simulink model "DBX_eARC_20220411_1632"  (R2021a)
settings: Solver=FixedStepAuto  StartTime=0.0  StopTime=inf  FixedStep=Ts  RelTol=1e-3  EnableMultiTasking=on
undefined symbols (not defined in the file): a, b, Cq, DiscIntNeverNeededParam, F_damper, Ff_spring, Fr_spring, FzF_0_w, FzR_0_w, h_CoG, h_RC, hs, hu, Ix, Iz, Kq, Kt, M, M_damp_f, M_damp_r, Mf_stiff, Mr_stiff, ms, mu, mui, params, theta_dot_f_damp, theta_dot_r_damp, theta_f_stiff, theta_r_stiff, tw, v_damper, Z_spring
libraries: CarMaker4SL x37, simulink_extras x1, simulink x1
(part 2 of 3)

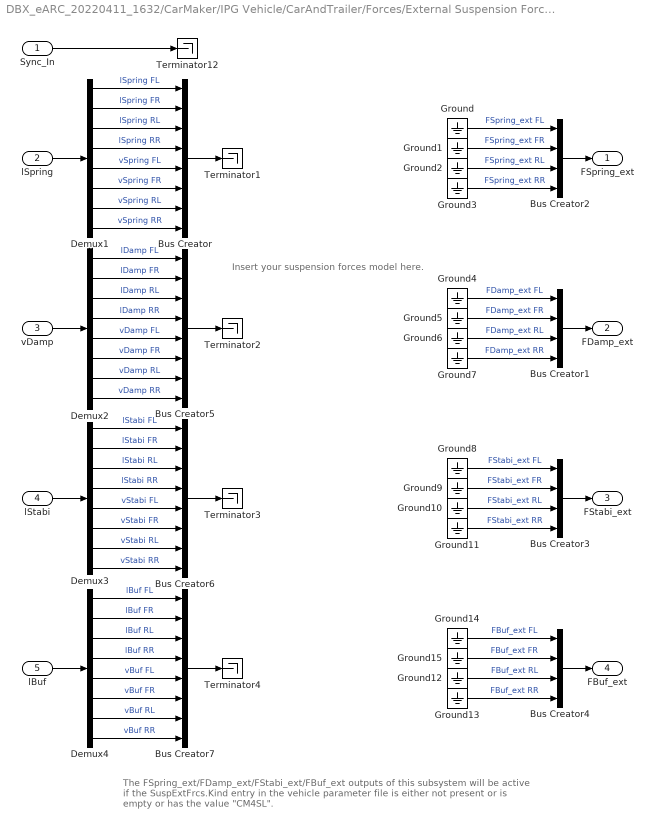
== system DBX_eARC_20220411_1632/CarMaker/IPG Vehicle/CarAndTrailer/Forces/External Suspension Forces ==
  note: The FSpring_ext/FDamp_ext/FStabi_ext/FBuf_ext outputs of this subsystem will be
      | active if the SuspExtFrcs.Kind entry in the vehicle parameter file
      | is either not present or is empty or has the value "CM4SL".
  note: Insert your suspension forces model here.
  Sync_In : Inport
  lSpring : Inport  Port=2
  vDamp : Inport  Port=3
  lStabi : Inport  Port=4
  lBuf : Inport  Port=5
  Bus Creator{,5..7} (4 alike) : BusCreator  Inputs=8
  Bus Creator{1..4} (4 alike) : BusCreator  Inputs=4
  Demux{1..4} (4 alike) : Demux  Outputs=8
      settings: DisplayOption=none
  Ground{,1..15} (16 alike) : Ground
  Terminator{1..4,12} (5 alike) : Terminator
  FSpring_ext : Outport
  FDamp_ext : Outport  Port=2
  FStabi_ext : Outport  Port=3
  FBuf_ext : Outport  Port=4
  wires:
  Bus Creator7/1 -> Terminator4/1
  Bus Creator6/1 -> Terminator3/1
  Bus Creator5/1 -> Terminator2/1
  Bus Creator/1 -> Terminator1/1
  Demux4/8 -> Bus Creator7/8  "vBuf RR"
  Demux4/7 -> Bus Creator7/7  "vBuf RL"
  Demux4/6 -> Bus Creator7/6  "vBuf FR"
  Demux4/5 -> Bus Creator7/5  "vBuf FL"
  Demux3/8 -> Bus Creator6/8  "vStabi RR"
  Demux3/7 -> Bus Creator6/7  "vStabi RL"
  Demux3/6 -> Bus Creator6/6  "vStabi FR"
  Demux3/5 -> Bus Creator6/5  "vStabi FL"
  Demux2/8 -> Bus Creator5/8  "vDamp RR"
  Demux2/7 -> Bus Creator5/7  "vDamp RL"
  Demux2/6 -> Bus Creator5/6  "vDamp FR"
  Demux2/5 -> Bus Creator5/5  "vDamp FL"
  Demux1/8 -> Bus Creator/8  "vSpring RR"
  Demux1/7 -> Bus Creator/7  "vSpring RL"
  Demux1/6 -> Bus Creator/6  "vSpring FR"
  Demux1/5 -> Bus Creator/5  "vSpring FL"
  Demux2/4 -> Bus Creator5/4  "lDamp RR"
  Demux2/3 -> Bus Creator5/3  "lDamp RL"
  Demux2/2 -> Bus Creator5/2  "lDamp FR"
  Demux2/1 -> Bus Creator5/1  "lDamp FL"
  Demux1/4 -> Bus Creator/4  "lSpring RR"
  Demux1/3 -> Bus Creator/3  "lSpring RL"
  Demux1/2 -> Bus Creator/2  "lSpring FR"
  Demux1/1 -> Bus Creator/1  "lSpring FL"
  Demux3/4 -> Bus Creator6/4  "lStabi RR"
  Demux3/3 -> Bus Creator6/3  "lStabi RL"
  Demux3/2 -> Bus Creator6/2  "lStabi FR"
  Demux3/1 -> Bus Creator6/1  "lStabi FL"
  lStabi/1 -> Demux3/1
  vDamp/1 -> Demux2/1
  lSpring/1 -> Demux1/1
  Demux4/4 -> Bus Creator7/4  "lBuf RR"
  Demux4/3 -> Bus Creator7/3  "lBuf RL"
  Demux4/2 -> Bus Creator7/2  "lBuf FR"
  Demux4/1 -> Bus Creator7/1  "lBuf FL"
  lBuf/1 -> Demux4/1
  Ground14/1 -> Bus Creator4/1  "FBuf_ext FL"
  Ground15/1 -> Bus Creator4/2  "FBuf_ext FR"
  Ground12/1 -> Bus Creator4/3  "FBuf_ext RL"
  Ground13/1 -> Bus Creator4/4  "FBuf_ext RR"
  Bus Creator4/1 -> FBuf_ext/1
  Sync_In/1 -> Terminator12/1
  Bus Creator2/1 -> FSpring_ext/1
  Ground/1 -> Bus Creator2/1  "FSpring_ext FL"
  Ground1/1 -> Bus Creator2/2  "FSpring_ext FR"
  Ground2/1 -> Bus Creator2/3  "FSpring_ext RL"
  Ground3/1 -> Bus Creator2/4  "FSpring_ext RR"
  Ground4/1 -> Bus Creator1/1  "FDamp_ext FL"
  Ground5/1 -> Bus Creator1/2  "FDamp_ext FR"
  Ground6/1 -> Bus Creator1/3  "FDamp_ext RL"
  Ground7/1 -> Bus Creator1/4  "FDamp_ext RR"
  Bus Creator1/1 -> FDamp_ext/1
  Ground8/1 -> Bus Creator3/1  "FStabi_ext FL"
  Ground9/1 -> Bus Creator3/2  "FStabi_ext FR"
  Ground10/1 -> Bus Creator3/3  "FStabi_ext RL"
  Ground11/1 -> Bus Creator3/4  "FStabi_ext RR"
  Bus Creator3/1 -> FStabi_ext/1

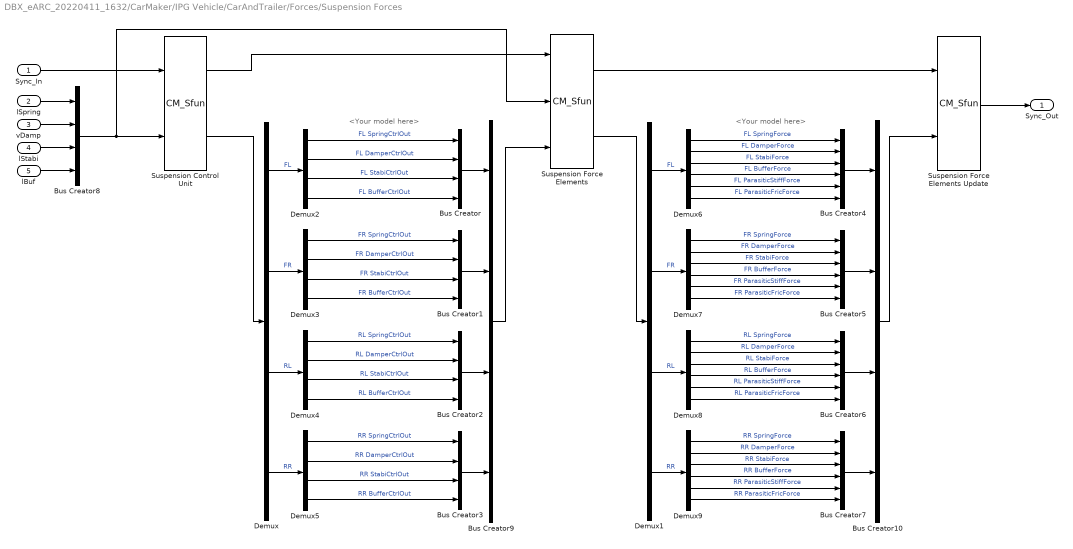
== system DBX_eARC_20220411_1632/CarMaker/IPG Vehicle/CarAndTrailer/Forces/Suspension Forces ==
  note: <Your model here>
  note: <Your model here>
  Sync_In : Inport
  lSpring : Inport  Port=2
  vDamp : Inport  Port=3
  lStabi : Inport  Port=4
  lBuf : Inport  Port=5
  Bus Creator{,1..3,8..10} (7 alike) : BusCreator  Inputs=4
  Bus Creator{4..7} (4 alike) : BusCreator  Inputs=6
  Demux{,1..5} (6 alike) : Demux
  Demux{6..9} (4 alike) : Demux  Outputs=6
  Suspension Control Unit : S-Function  FunctionName=CM_Sfun  Parameters='ForcesSuspControl'  SFunctionDeploymentMode=off  EnableBusSupport=off
  Suspension Force Elements : S-Function  FunctionName=CM_Sfun  Parameters='ForcesSusp'  SFunctionDeploymentMode=off  EnableBusSupport=off
  Suspension Force Elements Update : S-Function  FunctionName=CM_Sfun  Parameters='ForcesSuspUpd'  SFunctionDeploymentMode=off  EnableBusSupport=off
  Sync_Out : Outport
  wires:
  vDamp/1 -> Bus Creator8/2
  lStabi/1 -> Bus Creator8/3
  lBuf/1 -> Bus Creator8/4
  lSpring/1 -> Bus Creator8/1
  Bus Creator8/1 -> Suspension Control Unit/2, Suspension Force Elements/2
  Sync_In/1 -> Suspension Control Unit/1
  Suspension Control Unit/1 -> Suspension Force Elements/1
  Suspension Force Elements/1 -> Suspension Force Elements Update/1
  Suspension Force Elements Update/1 -> Sync_Out/1
  Bus Creator4/1 -> Bus Creator10/1
  Bus Creator5/1 -> Bus Creator10/2
  Bus Creator6/1 -> Bus Creator10/3
  Bus Creator7/1 -> Bus Creator10/4
  Demux6/1 -> Bus Creator4/1  "FL SpringForce"
  Demux9/1 -> Bus Creator7/1  "RR SpringForce"
  Demux9/2 -> Bus Creator7/2  "RR DamperForce"
  Demux9/3 -> Bus Creator7/3  "RR StabiForce"
  Demux9/4 -> Bus Creator7/4  "RR BufferForce"
  Demux9/5 -> Bus Creator7/5  "RR ParasiticStiffForce"
  Demux9/6 -> Bus Creator7/6  "RR ParasiticFricForce"
  Demux8/1 -> Bus Creator6/1  "RL SpringForce"
  Demux8/2 -> Bus Creator6/2  "RL DamperForce"
  Demux8/4 -> Bus Creator6/4  "RL BufferForce"
  Demux8/5 -> Bus Creator6/5  "RL ParasiticStiffForce"
  Demux8/6 -> Bus Creator6/6  "RL ParasiticFricForce"
  Demux8/3 -> Bus Creator6/3  "RL StabiForce"
  Demux7/1 -> Bus Creator5/1  "FR SpringForce"
  Demux7/2 -> Bus Creator5/2  "FR DamperForce"
  Demux7/3 -> Bus Creator5/3  "FR StabiForce"
  Demux7/4 -> Bus Creator5/4  "FR BufferForce"
  Demux7/5 -> Bus Creator5/5  "FR ParasiticStiffForce"
  Demux7/6 -> Bus Creator5/6  "FR ParasiticFricForce"
  Demux6/2 -> Bus Creator4/2  "FL DamperForce"
  Demux6/3 -> Bus Creator4/3  "FL StabiForce"
  Demux6/4 -> Bus Creator4/4  "FL BufferForce"
  Demux6/5 -> Bus Creator4/5  "FL ParasiticStiffForce"
  Demux6/6 -> Bus Creator4/6  "FL ParasiticFricForce"
  Bus Creator10/1 -> Suspension Force Elements Update/2
  Demux/1 -> Demux2/1  "FL"
  Bus Creator1/1 -> Bus Creator9/2
  Demux/2 -> Demux3/1  "FR"
  Bus Creator2/1 -> Bus Creator9/3
  Demux/3 -> Demux4/1  "RL"
  Bus Creator3/1 -> Bus Creator9/4
  Demux2/1 -> Bus Creator/1  "FL SpringCtrlOut"
  Demux/4 -> Demux5/1  "RR"
  Demux5/1 -> Bus Creator3/1  "RR SpringCtrlOut"
  Demux5/2 -> Bus Creator3/2  "RR DamperCtrlOut"
  Demux5/3 -> Bus Creator3/3  "RR StabiCtrlOut"
  Demux5/4 -> Bus Creator3/4  "RR BufferCtrlOut"
  Demux4/1 -> Bus Creator2/1  "RL SpringCtrlOut"
  Demux4/2 -> Bus Creator2/2  "RL DamperCtrlOut"
  Demux4/4 -> Bus Creator2/4  "RL BufferCtrlOut"
  Demux4/3 -> Bus Creator2/3  "RL StabiCtrlOut"
  Demux3/1 -> Bus Creator1/1  "FR SpringCtrlOut"
  Demux3/2 -> Bus Creator1/2  "FR DamperCtrlOut"
  Demux3/3 -> Bus Creator1/3  "FR StabiCtrlOut"
  Demux3/4 -> Bus Creator1/4  "FR BufferCtrlOut"
  Demux2/2 -> Bus Creator/2  "FL DamperCtrlOut"
  Demux2/3 -> Bus Creator/3  "FL StabiCtrlOut"
  Demux2/4 -> Bus Creator/4  "FL BufferCtrlOut"
  Suspension Control Unit/2 -> Demux/1
  Bus Creator9/1 -> Suspension Force Elements/3
  Bus Creator/1 -> Bus Creator9/1
  Suspension Force Elements/2 -> Demux1/1
  Demux1/1 -> Demux6/1  "FL"
  Demux1/2 -> Demux7/1  "FR"
  Demux1/3 -> Demux8/1  "RL"
  Demux1/4 -> Demux9/1  "RR"

== system DBX_eARC_20220411_1632/CarMaker/IPG Vehicle/CarAndTrailer/Forces/Tires ==
  note: The TireXX_Out signals will only be used if FileIdent is "CarMaker-Tire-CM4SL" in the tire parameter file!
      | An example parameter file can be found in Data/Tire/DT_CM4SL_UserTire.
  Sync_In : Inport
  TireFL_In : Inport  Port=2
  TireFR_In : Inport  Port=3
  TireRL_In : Inport  Port=4
  TireRR_In : Inport  Port=5
  Bus Creator{1..4} (4 alike) : BusCreator  Inputs=11
  Demux{1..3,8} (4 alike) : Demux  Outputs=7
      settings: DisplayOption=none
  TireFL : Subsystem
  TireFR : Subsystem
  TireRL : Subsystem
  TireRR : Subsystem
  TireFL_Out : Outport
  TireFR_Out : Outport  Port=2
  TireRL_Out : Outport  Port=3
  TireRR_Out : Outport  Port=4
  wires:
  Sync_In/1 -> TireRR/1(Sync_In), TireRL/1(Sync_In), TireFR/1(Sync_In), TireFL/1(Sync_In)
  Bus Creator4/1 -> TireRR_Out/1
  Bus Creator2/1 -> TireRL_Out/1
  Bus Creator1/1 -> TireFR_Out/1
  Demux3/5 -> TireRR/6(Rim_turnv)  "Tire_In Rim_turnv"
  Demux3/4 -> TireRR/5(Rim_rotv)  "Tire_In Rim_rotv"
  Demux3/1 -> TireRR/2(Load)  "Tire_In Load"
  Demux3/7 -> TireRR/8(muRoad)  "Tire_In mu"
  Demux3/6 -> TireRR/7(InclinAngle)  "Tire_In Camber"
  Demux3/2 -> TireRR/3(vxtrans)  "Tire_In vxtrans"
  Demux3/3 -> TireRR/4(vytrans)  "Tire_In vytrans"
  TireRR/11(AlignTrq) -> Bus Creator4/11  "Tire_Out AlignTrq"
  TireRR/10(RollResist) -> Bus Creator4/10  "Tire_Out RollResist"
  TireRR/9(OverturnTrq) -> Bus Creator4/9  "Tire_Out OverturnTrq"
  TireRR/8(LoadFrc) -> Bus Creator4/8  "Tire_Out LoadFrc"
  TireRR/7(SideFrc) -> Bus Creator4/7  "Tire_Out SideFrc"
  TireRR/6(LongFrc) -> Bus Creator4/6  "Tire_Out LongFrc"
  TireRR/5(vBelt) -> Bus Creator4/5  "Tire_Out vBelt"
  TireRR/4(rBelt_eff) -> Bus Creator4/4  "Tire_Out rBelt_eff"
  TireRR/3(TurnSlp) -> Bus Creator4/3  "Tire_Out TurnSlp"
  TireRR/1(Slp) -> Bus Creator4/1  "Tire_Out Slp"
  TireRR/2(Alpha) -> Bus Creator4/2  "Tire_Out Alpha"
  Demux2/5 -> TireRL/6(Rim_turnv)  "Tire_In Rim_turnv"
  Demux2/4 -> TireRL/5(Rim_rotv)  "Tire_In Rim_rotv"
  Demux2/1 -> TireRL/2(Load)  "Tire_In Load"
  Demux2/7 -> TireRL/8(muRoad)  "Tire_In mu"
  Demux2/6 -> TireRL/7(InclinAngle)  "Tire_In Camber"
  Demux2/2 -> TireRL/3(vxtrans)  "Tire_In vxtrans"
  Demux2/3 -> TireRL/4(vytrans)  "Tire_In vytrans"
  TireRL/11(AlignTrq) -> Bus Creator2/11  "Tire_Out AlignTrq"
  TireRL/10(RollResist) -> Bus Creator2/10  "Tire_Out RollResist"
  TireRL/9(OverturnTrq) -> Bus Creator2/9  "Tire_Out OverturnTrq"
  TireRL/8(LoadFrc) -> Bus Creator2/8  "Tire_Out LoadFrc"
  TireRL/7(SideFrc) -> Bus Creator2/7  "Tire_Out SideFrc"
  TireRL/6(LongFrc) -> Bus Creator2/6  "Tire_Out LongFrc"
  TireRL/5(vBelt) -> Bus Creator2/5  "Tire_Out vBelt"
  TireRL/4(rBelt_eff) -> Bus Creator2/4  "Tire_Out rBelt_eff"
  TireRL/3(TurnSlp) -> Bus Creator2/3  "Tire_Out TurnSlp"
  TireRL/1(Slp) -> Bus Creator2/1  "Tire_Out Slp"
  TireRL/2(Alpha) -> Bus Creator2/2  "Tire_Out Alpha"
  Demux1/5 -> TireFR/6(Rim_turnv)  "Tire_In Rim_turnv"
  Demux1/4 -> TireFR/5(Rim_rotv)  "Tire_In Rim_rotv"
  Demux1/1 -> TireFR/2(Load)  "Tire_In Load"
  Demux1/7 -> TireFR/8(muRoad)  "Tire_In mu"
  Demux1/6 -> TireFR/7(InclinAngle)  "Tire_In Camber"
  Demux1/2 -> TireFR/3(vxtrans)  "Tire_In vxtrans"
  Demux1/3 -> TireFR/4(vytrans)  "Tire_In vytrans"
  TireFR/11(AlignTrq) -> Bus Creator1/11  "Tire_Out AlignTrq"
  TireFR/10(RollResist) -> Bus Creator1/10  "Tire_Out RollResist"
  TireFR/9(OverturnTrq) -> Bus Creator1/9  "Tire_Out OverturnTrq"
  TireFR/8(LoadFrc) -> Bus Creator1/8  "Tire_Out LoadFrc"
  TireFR/7(SideFrc) -> Bus Creator1/7  "Tire_Out SideFrc"
  TireFR/6(LongFrc) -> Bus Creator1/6  "Tire_Out LongFrc"
  TireFR/5(vBelt) -> Bus Creator1/5  "Tire_Out vBelt"
  TireFR/4(rBelt_eff) -> Bus Creator1/4  "Tire_Out rBelt_eff"
  TireFR/3(TurnSlp) -> Bus Creator1/3  "Tire_Out TurnSlp"
  TireFR/1(Slp) -> Bus Creator1/1  "Tire_Out Slp"
  TireFR/2(Alpha) -> Bus Creator1/2  "Tire_Out Alpha"
  Demux8/5 -> TireFL/6(Rim_turnv)  "Tire_In Rim_turnv"
  Demux8/4 -> TireFL/5(Rim_rotv)  "Tire_In Rim_rotv"
  TireFL_In/1 -> Demux8/1
  Demux8/1 -> TireFL/2(Load)  "Tire_In Load"
  Demux8/7 -> TireFL/8(muRoad)  "Tire_In mu"
  Demux8/6 -> TireFL/7(InclinAngle)  "Tire_In Camber"
  Demux8/2 -> TireFL/3(vxtrans)  "Tire_In vxtrans"
  Demux8/3 -> TireFL/4(vytrans)  "Tire_In vytrans"
  TireFL/11(AlignTrq) -> Bus Creator3/11  "Tire_Out AlignTrq"
  TireFL/10(RollResist) -> Bus Creator3/10  "Tire_Out RollResist"
  TireFL/9(OverturnTrq) -> Bus Creator3/9  "Tire_Out OverturnTrq"
  TireFL/8(LoadFrc) -> Bus Creator3/8  "Tire_Out LoadFrc"
  TireFL/7(SideFrc) -> Bus Creator3/7  "Tire_Out SideFrc"
  TireFL/6(LongFrc) -> Bus Creator3/6  "Tire_Out LongFrc"
  TireFL/5(vBelt) -> Bus Creator3/5  "Tire_Out vBelt"
  TireFL/4(rBelt_eff) -> Bus Creator3/4  "Tire_Out rBelt_eff"
  TireFL/3(TurnSlp) -> Bus Creator3/3  "Tire_Out TurnSlp"
  TireFL/1(Slp) -> Bus Creator3/1  "Tire_Out Slp"
  TireFL/2(Alpha) -> Bus Creator3/2  "Tire_Out Alpha"
  Bus Creator3/1 -> TireFL_Out/1
  TireFR_In/1 -> Demux1/1
  TireRL_In/1 -> Demux2/1
  TireRR_In/1 -> Demux3/1

== system DBX_eARC_20220411_1632/CarMaker/IPG Vehicle/CarAndTrailer/Forces/Vehicle Forces ==
  Sync_In : Inport
  Bus Creator1 : BusCreator  Inputs=12
  Bus Creator8 : BusCreator  Inputs=16
  BusCreator1 : BusCreator  Inputs=4
  BusCreator2 : BusCreator  Inputs=9
  Demux : Demux  Outputs=16
      settings: DisplayOption=none
  Demux1 : Demux  Outputs=12
      settings: DisplayOption=none
  Demux2 : Demux  Outputs=13
      settings: DisplayOption=none
  Forces : S-Function  FunctionName=CM_Sfun  Parameters='Forces'  SFunctionDeploymentMode=off  EnableBusSupport=off
  Terminator : Terminator
  Sync_Out : Outport
  Car.Virtual : Outport  Port=2
  Car.Aero : Outport  Port=3
  Car.Load : Outport  Port=4
  wires:
  BusCreator1/1 -> Terminator/1  "Aero IF (in)"
  Demux2/13 -> BusCreator2/9  "car Aero Trq_1 z"
  Demux2/12 -> BusCreator2/8  "car Aero Trq_1 y"
  Demux2/11 -> BusCreator2/7  "car Aero Trq_1 x"
  Demux2/10 -> BusCreator2/6  "car Aero Frc_1 z"
  Demux2/9 -> BusCreator2/5  "car Aero Frc_1 y"
  Demux2/8 -> BusCreator2/4  "car Aero Frc_1 x"
  Demux2/7 -> BusCreator2/3  "car Aero PoA_1 z"
  Demux2/6 -> BusCreator2/2  "car Aero PoA_1 y"
  Demux2/5 -> BusCreator2/1  "car Aero PoA_1 x"
  Demux2/4 -> BusCreator1/4  "car Aero tau_1"
  Demux2/3 -> BusCreator1/3  "car Aero ApproachVel_1 z"
  Demux2/2 -> BusCreator1/2  "car Aero ApproachVel_1 y"
  Demux2/1 -> BusCreator1/1  "car Aero ApproachVel_1 x"
  Demux/16 -> Bus Creator8/16  "Car Load_3 tz"
  Demux/15 -> Bus Creator8/15  "Car Load_3 ty"
  Demux/14 -> Bus Creator8/14  "Car Load_3 tx"
  Demux/13 -> Bus Creator8/13  "Car Load_3 mass"
  Demux1/12 -> Bus Creator1/12  "Car Virtual Trq_0 z"
  Demux1/11 -> Bus Creator1/11  "Car Virtual Trq_0 y"
  Demux1/10 -> Bus Creator1/10  "Car Virtual Trq_0 x"
  Demux1/9 -> Bus Creator1/9  "Car Virtual Trq_1 z"
  Demux1/8 -> Bus Creator1/8  "Car Virtual Trq_1 y"
  Demux1/7 -> Bus Creator1/7  "Car Virtual Trq_1 x"
  Demux1/6 -> Bus Creator1/6  "Car Virtual Frc_0 z"
  Demux1/5 -> Bus Creator1/5  "Car Virtual Frc_0 y"
  Demux1/4 -> Bus Creator1/4  "Car Virtual Frc_0 x"
  Sync_In/1 -> Forces/1
  Forces/1 -> Sync_Out/1
  BusCreator2/1 -> Car.Aero/1
  Demux1/1 -> Bus Creator1/1  "Car Virtual Frc_1 x"
  Demux1/2 -> Bus Creator1/2  "Car Virtual Frc_1 y"
  Demux1/3 -> Bus Creator1/3  "Car Virtual Frc_1 z"
  Forces/3 -> Demux2/1
  Forces/2 -> Demux1/1
  Bus Creator1/1 -> Car.Virtual/1
  Bus Creator8/1 -> Car.Load/1
  Demux/1 -> Bus Creator8/1  "Car Load_0 mass"
  Demux/2 -> Bus Creator8/2  "Car Load_0 tx"
  Demux/3 -> Bus Creator8/3  "Car Load_0 ty"
  Demux/4 -> Bus Creator8/4  "Car Load_0 tz"
  Demux/5 -> Bus Creator8/5  "Car Load_1 mass"
  Demux/6 -> Bus Creator8/6  "Car Load_1 tx"
  Demux/7 -> Bus Creator8/7  "Car Load_1 ty"
  Demux/8 -> Bus Creator8/8  "Car Load_1 tz"
  Demux/9 -> Bus Creator8/9  "Car Load_2 mass"
  Demux/10 -> Bus Creator8/10  "Car Load_2 tx"
  Demux/11 -> Bus Creator8/11  "Car Load_2 ty"
  Demux/12 -> Bus Creator8/12  "Car Load_2 tz"
  Forces/4 -> Demux/1

== system DBX_eARC_20220411_1632/CarMaker/IPG Vehicle/CarAndTrailer/Trailer/Averaging Slip Angle in rads ==
  In1 : Inport
  In2 : Inport  Port=2
  In3 : Inport  Port=3
  In4 : Inport  Port=4
  Add : Sum  Inputs=4
  Bus Selector10 : BusSelector  OutputSignals=Vhcl Wheel RR SideSlip
  Bus Selector7 : BusSelector  OutputSignals=Vhcl Wheel FL SideSlip
  Bus Selector8 : BusSelector  OutputSignals=Vhcl Wheel FR SideSlip
  Bus Selector9 : BusSelector  OutputSignals=Vhcl Wheel RL SideSlip
  Gain2 : Gain  Gain=1/4
  Out1 : Outport
  wires:
  Bus Selector10/1 -> Add/4  "<Vhcl Wheel RR SideSlip>"
  In4/1 -> Bus Selector10/1
  Gain2/1 -> Out1/1
  Bus Selector7/1 -> Add/1  "<Vhcl Wheel FL SideSlip>"
  In1/1 -> Bus Selector7/1
  Bus Selector9/1 -> Add/3  "<Vhcl Wheel RL SideSlip>"
  Add/1 -> Gain2/1
  Bus Selector8/1 -> Add/2  "<Vhcl Wheel FR SideSlip>"
  In2/1 -> Bus Selector8/1
  In3/1 -> Bus Selector9/1

== system DBX_eARC_20220411_1632/CarMaker/IPG Vehicle/CarAndTrailer/Trailer/CreateBus Car.Hitch.FrcTrq ==
  In1 : Inport
  Bus Creator7 : BusCreator  Inputs=6
  Demux7 : Demux  Outputs=6
      settings: DisplayOption=none
  Out1 : Outport
  wires:
  In1/1 -> Demux7/1
  Bus Creator7/1 -> Out1/1
  Demux7/6 -> Bus Creator7/6  "Car Hitch Trq2Car z"
  Demux7/5 -> Bus Creator7/5  "Car Hitch Trq2Car y"
  Demux7/4 -> Bus Creator7/4  "Car Hitch Trq2Car x"
  Demux7/3 -> Bus Creator7/3  "Car Hitch Frc2Car z"
  Demux7/2 -> Bus Creator7/2  "Car Hitch Frc2Car y"
  Demux7/1 -> Bus Creator7/1  "Car Hitch Frc2Car x"

== system DBX_eARC_20220411_1632/CarMaker/IPG Vehicle/CarAndTrailer/Trailer/CreateBus Vhcl.Motion ==
  note: Integrated Roll Angle Needs Correction from Roll Angle calculation based on Ride Height Sensor Measurement
  In1 : Inport
  Bus Selector : BusSelector  OutputSignals=Vhcl RollAcc,Vhcl RollVel,Vhcl Roll
  BusCreator : BusCreator  Inputs=15
  Demux : Demux  Outputs=15
      settings: DisplayOption=none
  Discrete-Time Integrator : DiscreteIntegrator  SampleTime=20e-3  ICPrevOutput=DiscIntNeverNeededParam  ICPrevScaledInput=DiscIntNeverNeededParam
  Discrete-Time Integrator1 : DiscreteIntegrator  SampleTime=20e-3  ICPrevOutput=DiscIntNeverNeededParam  ICPrevScaledInput=DiscIntNeverNeededParam
  Integrator : Integrator
  Integrator1 : Integrator
  Mux : Mux  Inputs=3
  Mux1 : Mux  Inputs=3
  Rate Transition : RateTransition  OutPortSampleTime=20e-3
  Rate Transition1 : RateTransition
  Rate Transition2 : RateTransition
  Scope : Scope
  Scope1 : Scope  NumInputPorts=3
  Out1 : Outport
  wires:
  Demux/15 -> BusCreator/15  "Vhcl YawAcc"
  Demux/14 -> BusCreator/14  "Vhcl YawVel"
  Demux/13 -> BusCreator/13  "Vhcl Yaw"
  Demux/12 -> BusCreator/12  "Vhcl PitchAcc"
  Demux/11 -> BusCreator/11  "Vhcl PitchVel"
  Demux/10 -> BusCreator/10  "Vhcl Pitch"
  Demux/9 -> BusCreator/9  "Vhcl RollAcc"
  Demux/8 -> BusCreator/8  "Vhcl RollVel"
  Demux/7 -> BusCreator/7  "Vhcl Roll"
  Demux/6 -> BusCreator/6  "Vhcl Hitch_Pos z"
  Demux/5 -> BusCreator/5  "Vhcl Hitch_Pos y"
  Demux/4 -> BusCreator/4  "Vhcl Hitch_Pos x"
  Demux/3 -> BusCreator/3  "Vhcl sRoad"
  Demux/2 -> BusCreator/2  "Vhcl Distance"
  Demux/1 -> Scope/1, BusCreator/1  "Vhcl v"
  In1/1 -> Demux/1
  BusCreator/1 -> Bus Selector/1, Out1/1
  Bus Selector/1 -> Scope1/1, Integrator/1, Rate Transition/1  "<Vhcl RollAcc>"
  Integrator/1 -> Mux/3, Integrator1/1  "Vehicle RollVel"
  Integrator1/1 -> Mux1/3  "Roll Angle"
  Bus Selector/2 -> Mux/1  "<Vhcl RollVel>"
  Bus Selector/3 -> Mux1/1  "<Vhcl Roll>"
  Mux1/1 -> Scope1/3
  Mux/1 -> Scope1/2
  Discrete-Time Integrator/1 -> Discrete-Time Integrator1/1, Rate Transition2/1
  Discrete-Time Integrator1/1 -> Rate Transition1/1
  Rate Transition/1 -> Discrete-Time Integrator/1
  Rate Transition1/1 -> Mux1/2
  Rate Transition2/1 -> Mux/2

== system DBX_eARC_20220411_1632/CarMaker/IPG Vehicle/CarAndTrailer/Trailer/CreateBus Vhcl.PoI ==
  In1 : Inport
  Bus Creator3 : BusCreator  Inputs=18
  Demux3 : Demux  Outputs=18
      settings: DisplayOption=none
  Out1 : Outport
  wires:
  Demux3/18 -> Bus Creator3/18  "Vhcl PoI_GCS Elev"
  Demux3/17 -> Bus Creator3/17  "Vhcl PoI_GCS Lat"
  Demux3/16 -> Bus Creator3/16  "Vhcl PoI_GCS Long"
  Demux3/15 -> Bus Creator3/15  "Vhcl PoI_Acc_1 z"
  Demux3/14 -> Bus Creator3/14  "Vhcl PoI_Acc_1 y"
  Demux3/13 -> Bus Creator3/13  "Vhcl PoI_Acc_1 x"
  Demux3/12 -> Bus Creator3/12  "Vhcl PoI_Vel_1 z"
  Demux3/11 -> Bus Creator3/11  "Vhcl PoI_Vel_1 y"
  Demux3/10 -> Bus Creator3/10  "Vhcl PoI_Vel_1 x"
  Demux3/9 -> Bus Creator3/9  "Vhcl PoI_Acc z"
  Demux3/8 -> Bus Creator3/8  "Vhcl PoI_Acc y"
  Demux3/7 -> Bus Creator3/7  "Vhcl PoI_Acc x"
  Demux3/6 -> Bus Creator3/6  "Vhcl PoI_Vel z"
  Demux3/5 -> Bus Creator3/5  "Vhcl PoI_Vel y"
  Demux3/4 -> Bus Creator3/4  "Vhcl PoI_Vel x"
  Demux3/3 -> Bus Creator3/3  "Vhcl PoI_Pos z"
  Demux3/2 -> Bus Creator3/2  "Vhcl PoI_Pos y"
  In1/1 -> Demux3/1
  Bus Creator3/1 -> Out1/1
  Demux3/1 -> Bus Creator3/1  "Vhcl PoI_Pos x"

== system DBX_eARC_20220411_1632/CarMaker/IPG Vehicle/CarAndTrailer/Trailer/CreateBus Vhcl.Steering ==
  In1 : Inport
  Bus Creator3 : BusCreator  Inputs=4
  Demux : Demux
      settings: DisplayOption=none
  Out1 : Outport
  wires:
  Bus Creator3/1 -> Out1/1
  Demux/1 -> Bus Creator3/1  "Vhcl Steering Ang"
  Demux/3 -> Bus Creator3/3  "Vhcl Steering AngAcc"
  Demux/2 -> Bus Creator3/2  "Vhcl Steering AngVel"
  Demux/4 -> Bus Creator3/4  "Vhcl Steering Trq"
  In1/1 -> Demux/1

== system DBX_eARC_20220411_1632/CarMaker/IPG Vehicle/CarAndTrailer/Trailer/CreateBus Vhcl.Wheel.FL ==
  In1 : Inport
  Bus Creator3 : BusCreator  Inputs=14
  Demux3 : Demux  Outputs=14
      settings: DisplayOption=none
  Out1 : Outport
  wires:
  Demux3/14 -> Bus Creator3/14  "Vhcl Wheel FL Trq_WhlBearing"
  Demux3/13 -> Bus Creator3/13  "Vhcl Wheel FL Trq_T2W"
  Demux3/12 -> Bus Creator3/12  "Vhcl Wheel FL SideSlip"
  Demux3/11 -> Bus Creator3/11  "Vhcl Wheel FL LongSlip"
  Demux3/10 -> Bus Creator3/10  "Vhcl Wheel FL vBelt"
  Demux3/9 -> Bus Creator3/9  "Vhcl Wheel FL Fz"
  Demux3/8 -> Bus Creator3/8  "Vhcl Wheel FL Fy"
  Demux3/7 -> Bus Creator3/7  "Vhcl Wheel FL Fx"
  Demux3/6 -> Bus Creator3/6  "Vhcl Wheel FL r_zxy z"
  Demux3/5 -> Bus Creator3/5  "Vhcl Wheel FL r_zxy y"
  Demux3/4 -> Bus Creator3/4  "Vhcl Wheel FL r_zxy x"
  Demux3/3 -> Bus Creator3/3  "Vhcl Wheel FL t z"
  Demux3/2 -> Bus Creator3/2  "Vhcl Wheel FL t y"
  In1/1 -> Demux3/1
  Bus Creator3/1 -> Out1/1
  Demux3/1 -> Bus Creator3/1  "Vhcl Wheel FL t x"

== system DBX_eARC_20220411_1632/CarMaker/IPG Vehicle/CarAndTrailer/Trailer/CreateBus Vhcl.Wheel.FR ==
  In1 : Inport
  Bus Creator3 : BusCreator  Inputs=14
  Demux3 : Demux  Outputs=14
      settings: DisplayOption=none
  Out1 : Outport
  wires:
  Demux3/14 -> Bus Creator3/14  "Vhcl Wheel FR Trq_WhlBearing"
  Demux3/13 -> Bus Creator3/13  "Vhcl Wheel FR Trq_T2W"
  Demux3/12 -> Bus Creator3/12  "Vhcl Wheel FR SideSlip"
  Demux3/11 -> Bus Creator3/11  "Vhcl Wheel FR LongSlip"
  Demux3/10 -> Bus Creator3/10  "Vhcl Wheel FR vBelt"
  Demux3/9 -> Bus Creator3/9  "Vhcl Wheel FR Fz"
  Demux3/8 -> Bus Creator3/8  "Vhcl Wheel FR Fy"
  Demux3/7 -> Bus Creator3/7  "Vhcl Wheel FR Fx"
  Demux3/6 -> Bus Creator3/6  "Vhcl Wheel FR r_zxy z"
  Demux3/5 -> Bus Creator3/5  "Vhcl Wheel FR r_zxy y"
  Demux3/4 -> Bus Creator3/4  "Vhcl Wheel FR r_zxy x"
  Demux3/3 -> Bus Creator3/3  "Vhcl Wheel FR t z"
  Demux3/2 -> Bus Creator3/2  "Vhcl Wheel FR t y"
  In1/1 -> Demux3/1
  Bus Creator3/1 -> Out1/1
  Demux3/1 -> Bus Creator3/1  "Vhcl Wheel FR t x"

== system DBX_eARC_20220411_1632/CarMaker/IPG Vehicle/CarAndTrailer/Trailer/CreateBus Vhcl.Wheel.RL ==
  In1 : Inport
  Bus Creator3 : BusCreator  Inputs=14
  Demux3 : Demux  Outputs=14
      settings: DisplayOption=none
  Out1 : Outport
  wires:
  Demux3/14 -> Bus Creator3/14  "Vhcl Wheel RL Trq_WhlBearing"
  Demux3/13 -> Bus Creator3/13  "Vhcl Wheel RL Trq_T2W"
  Demux3/12 -> Bus Creator3/12  "Vhcl Wheel RL SideSlip"
  Demux3/11 -> Bus Creator3/11  "Vhcl Wheel RL LongSlip"
  Demux3/10 -> Bus Creator3/10  "Vhcl Wheel RL vBelt"
  Demux3/9 -> Bus Creator3/9  "Vhcl Wheel RL Fz"
  Demux3/8 -> Bus Creator3/8  "Vhcl Wheel RL Fy"
  Demux3/7 -> Bus Creator3/7  "Vhcl Wheel RL Fx"
  Demux3/6 -> Bus Creator3/6  "Vhcl Wheel RL r_zxy z"
  Demux3/5 -> Bus Creator3/5  "Vhcl Wheel RL r_zxy y"
  Demux3/4 -> Bus Creator3/4  "Vhcl Wheel RL r_zxy x"
  Demux3/3 -> Bus Creator3/3  "Vhcl Wheel RL t z"
  Demux3/2 -> Bus Creator3/2  "Vhcl Wheel RL t y"
  In1/1 -> Demux3/1
  Bus Creator3/1 -> Out1/1
  Demux3/1 -> Bus Creator3/1  "Vhcl Wheel RL t x"

== system DBX_eARC_20220411_1632/CarMaker/IPG Vehicle/CarAndTrailer/Trailer/CreateBus Vhcl.Wheel.RR ==
  In1 : Inport
  Bus Creator3 : BusCreator  Inputs=14
  Demux3 : Demux  Outputs=14
      settings: DisplayOption=none
  Out1 : Outport
  wires:
  Demux3/14 -> Bus Creator3/14  "Vhcl Wheel RR Trq_WhlBearing"
  Demux3/13 -> Bus Creator3/13  "Vhcl Wheel RR Trq_T2W"
  Demux3/12 -> Bus Creator3/12  "Vhcl Wheel RR SideSlip"
  Demux3/11 -> Bus Creator3/11  "Vhcl Wheel RR LongSlip"
  Demux3/10 -> Bus Creator3/10  "Vhcl Wheel RR vBelt"
  Demux3/9 -> Bus Creator3/9  "Vhcl Wheel RR Fz"
  Demux3/8 -> Bus Creator3/8  "Vhcl Wheel RR Fy"
  Demux3/7 -> Bus Creator3/7  "Vhcl Wheel RR Fx"
  Demux3/6 -> Bus Creator3/6  "Vhcl Wheel RR r_zxy z"
  Demux3/5 -> Bus Creator3/5  "Vhcl Wheel RR r_zxy y"
  Demux3/4 -> Bus Creator3/4  "Vhcl Wheel RR r_zxy x"
  Demux3/3 -> Bus Creator3/3  "Vhcl Wheel RR t z"
  Demux3/2 -> Bus Creator3/2  "Vhcl Wheel RR t y"
  In1/1 -> Demux3/1
  Bus Creator3/1 -> Out1/1
  Demux3/1 -> Bus Creator3/1  "Vhcl Wheel RR t x"

== system DBX_eARC_20220411_1632/CarMaker/IPG Vehicle/CarAndTrailer/Trailer/MIMO 4DOF roll with LT ==
  delta_deg : Inport
  u : Inport  Port=2
  T_ARB_f : Inport  Port=3
  T_ARB_r : Inport  Port=4
  x0 : Inport  Port=5
  4 DOF model : Subsystem
  Bicycle model : Subsystem
  Constant1 : Constant  Value=0
  Constant2 : Constant  Value=0
  Delay : Delay  DelayLength=1
  Demux : Demux  Outputs=10
  Demux1 : Demux  Outputs=8
  Gain2 : Gain
  Mux : Mux  Inputs=8
  Scope5 : Scope
  ay : Outport
  r_radps : Outport  Port=2
  r_dot_rad : Outport  Port=3
  phi : Outport  Port=4
  phi_dot : Outport  Port=5
  zc : Outport  Port=6
  zc_dot : Outport  Port=7
  Ku : Outport  Port=8
  wires:
  Demux/10 -> Mux/8
  Demux1/6 -> 4 DOF model/11(zu1_dot_0)
  u/1 -> Bicycle model/2(u)
  Gain2/1 -> Scope5/1, Bicycle model/1(delta_deg)  "delta_deg"
  Demux/6 -> Mux/4
  Demux1/8 -> 4 DOF model/13(zu2_dot_0)
  4 DOF model/6(Lt_r) -> Bicycle model/6(Lt_r)
  Demux1/7 -> 4 DOF model/12(zu2_0)
  Demux1/5 -> 4 DOF model/10(zu1_0)
  Demux1/3 -> 4 DOF model/8(phi_0)
  Bicycle model/3(r_dot_rad) -> r_dot_rad/1
  T_ARB_r/1 -> 4 DOF model/5(T_ARB_r)
  Demux/9 -> Mux/7
  Constant1/1 -> 4 DOF model/3(zr2)
  Constant2/1 -> 4 DOF model/2(zr1)
  delta_deg/1 -> Gain2/1
  Delay/1 -> ay/1, 4 DOF model/1(ay)  "ay"
  Demux/3 -> Mux/1
  Demux/5 -> Mux/3
  Mux/1 -> Demux1/1
  Demux1/2 -> 4 DOF model/7(zc_dot_0)
  Demux/7 -> Mux/5
  Bicycle model/4(Ku) -> Ku/1  "Ku"
  4 DOF model/2(phi_dot) -> phi_dot/1  "phi_dot"
  4 DOF model/5(Lt_f) -> Bicycle model/5(Lt_f)
  Demux/4 -> Mux/2
  Demux1/1 -> 4 DOF model/6(zc_0)
  Demux1/4 -> 4 DOF model/9(phi_dot_0)
  Demux/2 -> Bicycle model/4(r_0)  "r_0"
  Demux/8 -> Mux/6
  Demux/1 -> Bicycle model/3(v_0)  "v_0"
  Bicycle model/2(r_rad) -> r_radps/1  "r_rad"
  x0/1 -> Demux/1
  4 DOF model/4(zc_dot) -> zc_dot/1  "zc_dot"
  T_ARB_f/1 -> 4 DOF model/4(T_ARB_f)
  4 DOF model/3(zc) -> zc/1  "zc"
  4 DOF model/1(phi) -> phi/1  "phi"
  Bicycle model/1(ay) -> Delay/1  "ay"

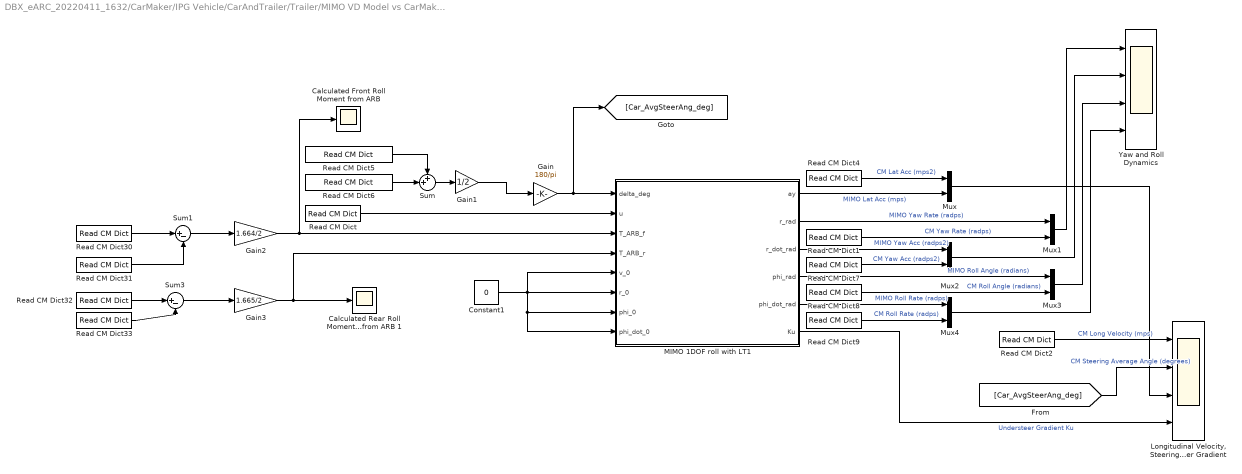
== system DBX_eARC_20220411_1632/CarMaker/IPG Vehicle/CarAndTrailer/Trailer/MIMO VD Model vs CarMaker ==
  "Calculated Front Roll Moment from ARB " : Scope
  Calculated Rear Roll Moment from ARB 1 : Scope
  Constant1 : Constant  Value=0
  Gain : Gain  Gain=180/pi
      settings: AttributesFormatString=Gain = %<Gain>
  Gain1 : Gain  Gain=1/2
  Gain2 : Gain  Gain=1.664/2
  Gain3 : Gain  Gain=1.665/2
  "Longitudinal Velocity, Steering Angle, Lateral Acceleration and Understeer Gradient" : Scope  NumInputPorts=4
  MIMO 1DOF roll with LT1 : Subsystem  TreatAsAtomicUnit=on
      settings: MinAlgLoopOccurrences=on
  Mux{,1..4} (5 alike) : Mux  Inputs=2
  Read CM Dict : CarMaker4SL/Read CM Dict  xname=Car.vx  xsync=off  xstime=Continuous
  Read CM Dict1 : CarMaker4SL/Read CM Dict  xname=Car.YawRate  xsync=off  xstime=Continuous
  Read CM Dict2 : CarMaker4SL/Read CM Dict  xname=Car.vx  xsync=off  xstime=Continuous
  Read CM Dict30 : CarMaker4SL/Read CM Dict  xname=Car.StabiFL.Frc  xsync=off  xstime=Continuous
  Read CM Dict31 : CarMaker4SL/Read CM Dict  xname=Car.StabiFR.Frc  xsync=off  xstime=Continuous
  Read CM Dict32 : CarMaker4SL/Read CM Dict  xname=Car.StabiRL.Frc  xsync=off  xstime=Continuous
  Read CM Dict33 : CarMaker4SL/Read CM Dict  xname=Car.StabiRR.Frc  xsync=off  xstime=Continuous
  Read CM Dict4 : CarMaker4SL/Read CM Dict  xname=Car.ay  xsync=off  xstime=Continuous
  Read CM Dict5 : CarMaker4SL/Read CM Dict  xname=Car.SteerAngleFL  xsync=off  xstime=Continuous
  Read CM Dict6 : CarMaker4SL/Read CM Dict  xname=Car.SteerAngleFR  xsync=off  xstime=Continuous
  Read CM Dict7 : CarMaker4SL/Read CM Dict  xname=Car.YawAcc  xsync=off  xstime=Continuous
  Read CM Dict8 : CarMaker4SL/Read CM Dict  xname=Car.Roll  xsync=off  xstime=Continuous
  Read CM Dict9 : CarMaker4SL/Read CM Dict  xname=Car.RollVel  xsync=off  xstime=Continuous
  Sum : Sum  Inputs=++|
  Sum1 : Sum  Inputs=|+-
  Sum3 : Sum  Inputs=|+-
  Yaw and Roll Dynamics : Scope  NumInputPorts=4
  wires:
  Sum1/1 -> Gain2/1
  Mux/1 -> "Longitudinal Velocity, Steering Angle, Lateral Acceleration and Understeer Gradient"/3
  MIMO 1DOF roll with LT1/1(ay) -> Mux/2  "MIMO Lat Acc (mps)"
  Read CM Dict7/1 -> Mux2/2  "CM Yaw Acc (radps2)"
  Read CM Dict32/1 -> Sum3/1
  Mux1/1 -> Yaw and Roll Dynamics/1
  Read CM Dict4/1 -> Mux/1  "CM Lat Acc (mps2)"
  Read CM Dict5/1 -> Sum/1
  Gain1/1 -> Gain/1
  Constant1/1 -> MIMO 1DOF roll with LT1/5(v_0), MIMO 1DOF roll with LT1/6(r_0), MIMO 1DOF roll with LT1/7(phi_0), MIMO 1DOF roll with LT1/8(phi_dot_0)
  Sum3/1 -> Gain3/1
  Read CM Dict30/1 -> Sum1/1
  MIMO 1DOF roll with LT1/2(r_rad) -> Mux1/1  "MIMO Yaw Rate (radps)"
  Read CM Dict31/1 -> Sum1/2
  Read CM Dict33/1 -> Sum3/2
  Read CM Dict8/1 -> Mux3/2  "CM Roll Angle (radians)"
  MIMO 1DOF roll with LT1/4(phi_rad) -> Mux3/1  "MIMO Roll Angle (radians)"
  Read CM Dict9/1 -> Mux4/2  "CM Roll Rate (radps)"
  Gain3/1 -> MIMO 1DOF roll with LT1/4(T_ARB_r), Calculated Rear Roll Moment from ARB 1/1
  MIMO 1DOF roll with LT1/3(r_dot_rad) -> Mux2/1  "MIMO Yaw Acc (radps2)"
  Sum/1 -> Gain1/1
  Read CM Dict6/1 -> Sum/2
  Gain2/1 -> MIMO 1DOF roll with LT1/3(T_ARB_f), "Calculated Front Roll Moment from ARB "/1
  Read CM Dict/1 -> MIMO 1DOF roll with LT1/2(u)
  Read CM Dict1/1 -> Mux1/2  "CM Yaw Rate (radps)"
  MIMO 1DOF roll with LT1/5(phi_dot_rad) -> Mux4/1  "MIMO Roll Rate (radps)"
  Mux4/1 -> Yaw and Roll Dynamics/4
  Mux3/1 -> Yaw and Roll Dynamics/3
  Gain/1 -> [Car_AvgSteerAng_deg], MIMO 1DOF roll with LT1/1(delta_deg)
  MIMO 1DOF roll with LT1/6(Ku) -> "Longitudinal Velocity, Steering Angle, Lateral Acceleration and Understeer Gradient"/4  "Understeer Gradient Ku"
  Mux2/1 -> Yaw and Roll Dynamics/2
  Read CM Dict2/1 -> "Longitudinal Velocity, Steering Angle, Lateral Acceleration and Understeer Gradient"/1  "CM Long Velocity (mps)"
  [Car_AvgSteerAng_deg] -> "Longitudinal Velocity, Steering Angle, Lateral Acceleration and Understeer Gradient"/2  "CM Steering Average Angle (degrees)"

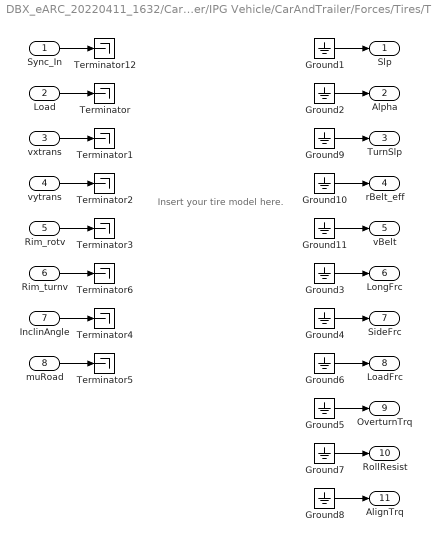
== system DBX_eARC_20220411_1632/CarMaker/IPG Vehicle/CarAndTrailer/Forces/Tires/TireFL ==
  note: Insert your tire model here.
  Sync_In : Inport
  Load : Inport  Port=2
  vxtrans : Inport  Port=3
  vytrans : Inport  Port=4
  Rim_rotv : Inport  Port=5
  Rim_turnv : Inport  Port=6
  InclinAngle : Inport  Port=7
  muRoad : Inport  Port=8
  Ground{1..11} (11 alike) : Ground
  Terminator{,1..6,12} (8 alike) : Terminator
  Slp : Outport
  Alpha : Outport  Port=2
  TurnSlp : Outport  Port=3
  rBelt_eff : Outport  Port=4
  vBelt : Outport  Port=5
  LongFrc : Outport  Port=6
  SideFrc : Outport  Port=7
  LoadFrc : Outport  Port=8
  OverturnTrq : Outport  Port=9
  RollResist : Outport  Port=10
  AlignTrq : Outport  Port=11
  wires:
  Ground11/1 -> vBelt/1
  Ground10/1 -> rBelt_eff/1
  Ground9/1 -> TurnSlp/1
  Rim_turnv/1 -> Terminator6/1
  Sync_In/1 -> Terminator12/1
  Ground2/1 -> Alpha/1
  Ground3/1 -> LongFrc/1
  Ground4/1 -> SideFrc/1
  Ground5/1 -> OverturnTrq/1
  vxtrans/1 -> Terminator1/1
  vytrans/1 -> Terminator2/1
  Rim_rotv/1 -> Terminator3/1
  InclinAngle/1 -> Terminator4/1
  muRoad/1 -> Terminator5/1
  Load/1 -> Terminator/1
  Ground1/1 -> Slp/1
  Ground6/1 -> LoadFrc/1
  Ground7/1 -> RollResist/1
  Ground8/1 -> AlignTrq/1

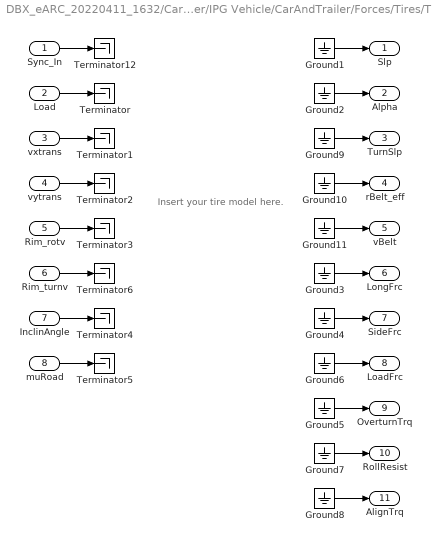
== system DBX_eARC_20220411_1632/CarMaker/IPG Vehicle/CarAndTrailer/Forces/Tires/TireFR ==
  note: Insert your tire model here.
  Sync_In : Inport
  Load : Inport  Port=2
  vxtrans : Inport  Port=3
  vytrans : Inport  Port=4
  Rim_rotv : Inport  Port=5
  Rim_turnv : Inport  Port=6
  InclinAngle : Inport  Port=7
  muRoad : Inport  Port=8
  Ground{1..11} (11 alike) : Ground
  Terminator{,1..6,12} (8 alike) : Terminator
  Slp : Outport
  Alpha : Outport  Port=2
  TurnSlp : Outport  Port=3
  rBelt_eff : Outport  Port=4
  vBelt : Outport  Port=5
  LongFrc : Outport  Port=6
  SideFrc : Outport  Port=7
  LoadFrc : Outport  Port=8
  OverturnTrq : Outport  Port=9
  RollResist : Outport  Port=10
  AlignTrq : Outport  Port=11
  wires:
  Ground11/1 -> vBelt/1
  Ground10/1 -> rBelt_eff/1
  Ground9/1 -> TurnSlp/1
  Rim_turnv/1 -> Terminator6/1
  Sync_In/1 -> Terminator12/1
  Ground2/1 -> Alpha/1
  Ground3/1 -> LongFrc/1
  Ground4/1 -> SideFrc/1
  Ground5/1 -> OverturnTrq/1
  vxtrans/1 -> Terminator1/1
  vytrans/1 -> Terminator2/1
  Rim_rotv/1 -> Terminator3/1
  InclinAngle/1 -> Terminator4/1
  muRoad/1 -> Terminator5/1
  Load/1 -> Terminator/1
  Ground1/1 -> Slp/1
  Ground6/1 -> LoadFrc/1
  Ground7/1 -> RollResist/1
  Ground8/1 -> AlignTrq/1

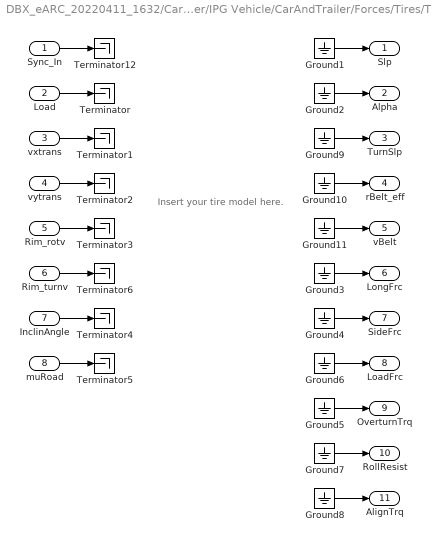
== system DBX_eARC_20220411_1632/CarMaker/IPG Vehicle/CarAndTrailer/Forces/Tires/TireRL ==
  note: Insert your tire model here.
  Sync_In : Inport
  Load : Inport  Port=2
  vxtrans : Inport  Port=3
  vytrans : Inport  Port=4
  Rim_rotv : Inport  Port=5
  Rim_turnv : Inport  Port=6
  InclinAngle : Inport  Port=7
  muRoad : Inport  Port=8
  Ground{1..11} (11 alike) : Ground
  Terminator{,1..6,12} (8 alike) : Terminator
  Slp : Outport
  Alpha : Outport  Port=2
  TurnSlp : Outport  Port=3
  rBelt_eff : Outport  Port=4
  vBelt : Outport  Port=5
  LongFrc : Outport  Port=6
  SideFrc : Outport  Port=7
  LoadFrc : Outport  Port=8
  OverturnTrq : Outport  Port=9
  RollResist : Outport  Port=10
  AlignTrq : Outport  Port=11
  wires:
  Ground11/1 -> vBelt/1
  Ground10/1 -> rBelt_eff/1
  Ground9/1 -> TurnSlp/1
  Rim_turnv/1 -> Terminator6/1
  Sync_In/1 -> Terminator12/1
  Ground2/1 -> Alpha/1
  Ground3/1 -> LongFrc/1
  Ground4/1 -> SideFrc/1
  Ground5/1 -> OverturnTrq/1
  vxtrans/1 -> Terminator1/1
  vytrans/1 -> Terminator2/1
  Rim_rotv/1 -> Terminator3/1
  InclinAngle/1 -> Terminator4/1
  muRoad/1 -> Terminator5/1
  Load/1 -> Terminator/1
  Ground1/1 -> Slp/1
  Ground6/1 -> LoadFrc/1
  Ground7/1 -> RollResist/1
  Ground8/1 -> AlignTrq/1

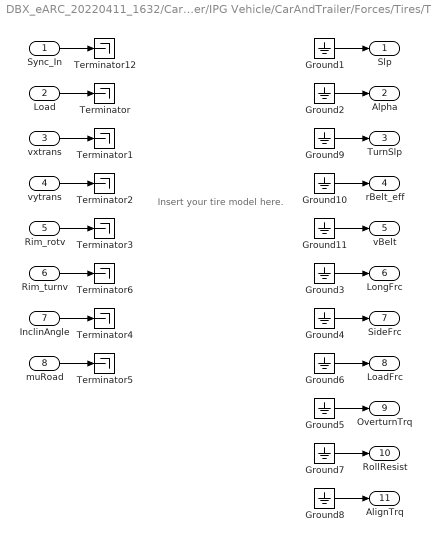
== system DBX_eARC_20220411_1632/CarMaker/IPG Vehicle/CarAndTrailer/Forces/Tires/TireRR ==
  note: Insert your tire model here.
  Sync_In : Inport
  Load : Inport  Port=2
  vxtrans : Inport  Port=3
  vytrans : Inport  Port=4
  Rim_rotv : Inport  Port=5
  Rim_turnv : Inport  Port=6
  InclinAngle : Inport  Port=7
  muRoad : Inport  Port=8
  Ground{1..11} (11 alike) : Ground
  Terminator{,1..6,12} (8 alike) : Terminator
  Slp : Outport
  Alpha : Outport  Port=2
  TurnSlp : Outport  Port=3
  rBelt_eff : Outport  Port=4
  vBelt : Outport  Port=5
  LongFrc : Outport  Port=6
  SideFrc : Outport  Port=7
  LoadFrc : Outport  Port=8
  OverturnTrq : Outport  Port=9
  RollResist : Outport  Port=10
  AlignTrq : Outport  Port=11
  wires:
  Ground11/1 -> vBelt/1
  Ground10/1 -> rBelt_eff/1
  Ground9/1 -> TurnSlp/1
  Rim_turnv/1 -> Terminator6/1
  Sync_In/1 -> Terminator12/1
  Ground2/1 -> Alpha/1
  Ground3/1 -> LongFrc/1
  Ground4/1 -> SideFrc/1
  Ground5/1 -> OverturnTrq/1
  vxtrans/1 -> Terminator1/1
  vytrans/1 -> Terminator2/1
  Rim_rotv/1 -> Terminator3/1
  InclinAngle/1 -> Terminator4/1
  muRoad/1 -> Terminator5/1
  Load/1 -> Terminator/1
  Ground1/1 -> Slp/1
  Ground6/1 -> LoadFrc/1
  Ground7/1 -> RollResist/1
  Ground8/1 -> AlignTrq/1

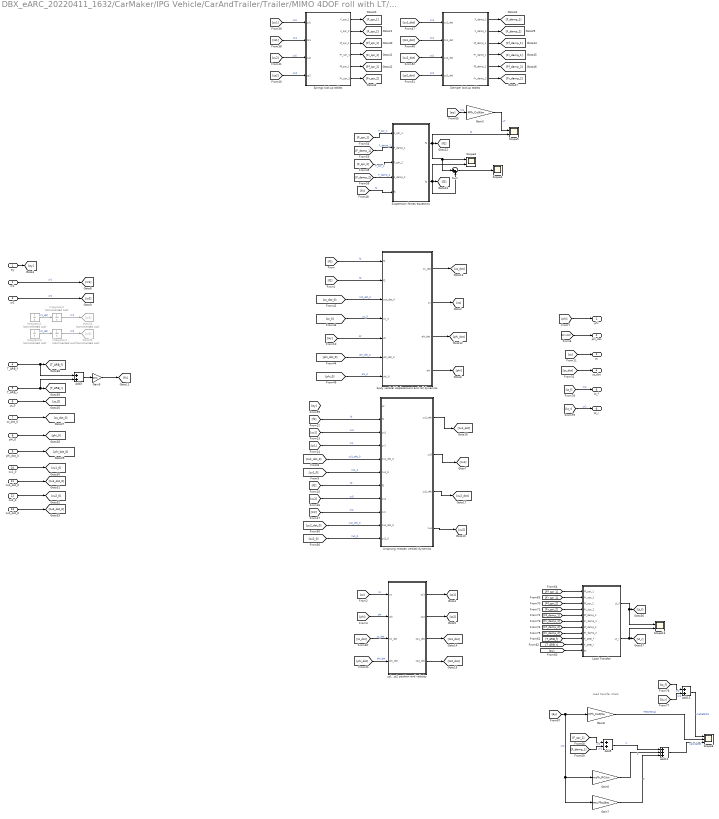
== system DBX_eARC_20220411_1632/CarMaker/IPG Vehicle/CarAndTrailer/Trailer/MIMO 4DOF roll with LT/4 DOF model ==
  note: Load transfer check
  ay : Inport
  zr1 : Inport  Port=2
  zr2 : Inport  Port=3
  T_ARB_f : Inport  Port=4
  T_ARB_r : Inport  Port=5
  zc_0 : Inport  Port=6
  zc_dot_0 : Inport  Port=7
  phi_0 : Inport  Port=8
  phi_dot_0 : Inport  Port=9
  zu1_0 : Inport  Port=10
  zu1_dot_0 : Inport  Port=11
  zu2_0 : Inport  Port=12
  zu2_dot_0 : Inport  Port=13
  Add12 : Sum  Inputs=+++
  Add13 : Sum
  Add3 : Sum
  Add5 : Sum
  Damper lookup tables : Subsystem
  Gain3 : Gain  Gain=M*h_CoG/tw
  Gain6 : Gain  Gain=ms*h_RC/tw
  Gain7 : Gain  Gain=mu*hu/tw
  Gain8 : Gain  Gain=M*h_CoG/tw
  Gain9 : Gain  Gain=1/tw
  Goto34 : Goto  Commented=on  GotoTag=zr1
  Goto35 : Goto  Commented=on  GotoTag=zr2
  Integrator{1..4} (4 alike) : Integrator  Commented=on
  Load Transfer : MATLAB Function  TreatAsAtomicUnit=on
  Scope13 : Scope  NumInputPorts=2
  Scope3 : Scope  NumInputPorts=2
  Scope4 : Scope
  Scope5 : Scope  NumInputPorts=2
  Scope6 : Scope  NumInputPorts=3
  Springs lookup tables : Subsystem
  Sum : Sum  Inputs=|++
  Suspension forces equations : Subsystem
  Unsprung masses vertical dynamics : Subsystem
  body vertical displacement and roll dynamics : Subsystem
  "zs1, zs2 position and velocity" : Subsystem
  phi : Outport
  phi_dot : Outport  Port=2
  zc : Outport  Port=3
  zc_dot : Outport  Port=4
  Lt_f : Outport  Port=5
  Lt_r : Outport  Port=6
  wires:
  [phi] -> phi/1
  ay/1 -> [ay]
  [zc] -> zc/1
  zr1/1 -> [zr1]  "zr1"
  zr2/1 -> [zr2]  "zr2"
  [phi_dot] -> phi_dot/1
  [zc_dot] -> zc_dot/1
  [zu1] -> Springs lookup tables/1(zu1)  "zu1"
  [zs1] -> Springs lookup tables/2(zs1)  "zs1"
  [zu2] -> Springs lookup tables/3(zu2)  "zu2"
  [zs2] -> Springs lookup tables/4(zs2)  "zs2"
  Springs lookup tables/1(F_spr_1) -> [F_spr_1]
  Springs lookup tables/2(F_spr_2) -> [F_spr_2]
  [zu1_dot] -> Damper lookup tables/1(zu1_dot)  "zu1"
  [zs2_dot] -> Damper lookup tables/4(zs2_dot)  "zs2"
  [zs1_dot] -> Damper lookup tables/2(zs1_dot)  "zs1"
  [zu2_dot] -> Damper lookup tables/3(zu2_dot)  "zu2"
  Damper lookup tables/1(F_damp_1) -> [F_damp_1]
  Damper lookup tables/2(F_damp_2) -> [F_damp_2]
  [F_spr_1] -> Suspension forces equations/1(F_spr_1)  "F_spr_1"
  [F_damp_1] -> Suspension forces equations/2(F_damp_1)  "F_damp_1"
  [F_spr_2] -> Suspension forces equations/3(F_spr_2)  "F_spr_2"
  [F_damp_2] -> Suspension forces equations/4(F_damp_2)  "F_damp_2"
  [fc] -> Suspension forces equations/5(fc)  "fc"
  Suspension forces equations/1(f1) -> Scope5/2, [f1], Sum/1, Scope3/1  "f1"
  Suspension forces equations/2(f2) -> Scope3/2, Sum/2, [f2]
  zc_0/1 -> [zc_0]
  zc_dot_0/1 -> [zc_dot_0]
  phi_dot_0/1 -> [phi_dot_0]
  phi_0/1 -> [phi_0]
  [f1] -> body vertical displacement and roll dynamics/1(f1)  "f1"
  [f2] -> body vertical displacement and roll dynamics/2(f2)  "f2"
  [zc_dot_0] -> body vertical displacement and roll dynamics/3(zct_dot_0)  "zct_dot_0"
  [zc_0] -> body vertical displacement and roll dynamics/4(zc_0)  "zc_0"
  [ay] -> body vertical displacement and roll dynamics/5(ay)  "ay"
  [phi_dot_0] -> body vertical displacement and roll dynamics/6(phi_dot_0)  "phi_dot_0"
  [phi_0] -> body vertical displacement and roll dynamics/7(phi_0)  "phi_0"
  body vertical displacement and roll dynamics/1(zc_dot) -> [zc_dot]
  body vertical displacement and roll dynamics/2(zc) -> [zc]
  body vertical displacement and roll dynamics/3(phi_dot) -> [phi_dot]
  body vertical displacement and roll dynamics/4(phi) -> [phi]
  zu1_0/1 -> [zu1_0]
  zu2_dot_0/1 -> [zu2_dot_0]
  zu2_0/1 -> [zu2_0]
  zu1_dot_0/1 -> [zu1_dot_0]
  [f1] -> Unsprung masses vertical dynamics/2(f1)  "f1"
  [zu1] -> Unsprung masses vertical dynamics/3(zu1)  "zu1"
  [zr1] -> Unsprung masses vertical dynamics/4(zr1)  "zr1"
  [zu1_dot_0] -> Unsprung masses vertical dynamics/5(zu1_dot_0)  "zu1_dot_0"
  [zu1_0] -> Unsprung masses vertical dynamics/6(zu1_0)  "zu1_0"
  [f2] -> Unsprung masses vertical dynamics/7(f2)  "f2"
  [zu2] -> Unsprung masses vertical dynamics/8(zu2)  "zu2"
  [zr2] -> Unsprung masses vertical dynamics/9(zr2)  "zr2"
  [zu2_dot_0] -> Unsprung masses vertical dynamics/10(zu2_dot_0)  "zu2_dot_0"
  [zu2_0] -> Unsprung masses vertical dynamics/11(zu2_0)  "zu2_0"
  Unsprung masses vertical dynamics/1(zu1_dot) -> [zu1_dot]
  Unsprung masses vertical dynamics/2(zu3) -> [zu1]
  Unsprung masses vertical dynamics/3(zu2_dot) -> [zu2_dot]
  Unsprung masses vertical dynamics/4(zu4) -> [zu2]
  [zc] -> "zs1, zs2 position and velocity"/1(zc)  "zc"
  [phi] -> "zs1, zs2 position and velocity"/2(phi)  "phi"
  [zc_dot] -> "zs1, zs2 position and velocity"/3(zc_dot)  "zc_dot"
  [phi_dot] -> "zs1, zs2 position and velocity"/4(phi_dot)  "phi_dot"
  "zs1, zs2 position and velocity"/1(zs1) -> [zs1]
  "zs1, zs2 position and velocity"/2(zs2) -> [zs2]
  "zs1, zs2 position and velocity"/3(zs1_dot) -> [zs1_dot]
  "zs1, zs2 position and velocity"/4(zs2_dot) -> [zs2_dot]
  Integrator2/1 -> Goto34/1  "zr1"
  Integrator4/1 -> Goto35/1  "zr2"
  Integrator3/1 -> Integrator4/1  "zr2_dot"
  Integrator1/1 -> Integrator2/1  "zr1_dot"
  Gain9/1 -> [fc]
  T_ARB_f/1 -> Add3/1, [T_ARB_f]
  T_ARB_r/1 -> Add3/2, [T_ARB_r]
  Add3/1 -> Gain9/1
  Sum/1 -> Scope4/1
  [ay] -> Gain3/1  "zr2"
  Gain3/1 -> Scope5/1  "LT"
  Springs lookup tables/3(Ff_spr_1) -> [Ff_spr_1]
  Springs lookup tables/4(Fr_spr_1) -> [Fr_spr_1]
  Springs lookup tables/5(Ff_spr_2) -> [Ff_spr_2]
  Springs lookup tables/6(Fr_spr_2) -> [Fr_spr_2]
  [F_spr_1] -> Add5/1  "zr2"
  [F_damp_1] -> Add5/2  "zr2"
  Add5/1 -> Add12/1  "1"
  [ay] -> Gain8/1, Gain7/1, Gain6/1  "zr2"
  Gain6/1 -> Add12/2  "2"
  Gain7/1 -> Add12/3  "3"
  Add12/1 -> Scope6/3  "calculated"
  Gain8/1 -> Scope6/2  "Theoretical"
  [Ff_spr_1] -> Load Transfer/1(Ff_spr_1)
  [T_ARB_r] -> Load Transfer/10(T_ARB_r)
  [Fr_spr_1] -> Load Transfer/2(Fr_spr_1)
  [T_ARB_f] -> Load Transfer/9(T_ARB_f)
  Load Transfer/1(Lt_f) -> Scope13/1, [Lt_f]
  [ay] -> Load Transfer/11(ay)
  Load Transfer/2(Lt_r) -> Scope13/2, [Lt_r]
  Damper lookup tables/3(Ff_damp_1) -> [Ff_damp_1]
  Damper lookup tables/4(Fr_damp_1) -> [Fr_damp_1]
  Damper lookup tables/5(Ff_damp_2) -> [Ff_damp_2]
  Damper lookup tables/6(Fr_damp_2) -> [Fr_damp_2]
  [Ff_spr_2] -> Load Transfer/3(Ff_spr_2)
  [Fr_spr_2] -> Load Transfer/4(Fr_spr_2)
  [Ff_damp_1] -> Load Transfer/5(Ff_damp_1)
  [Fr_damp_1] -> Load Transfer/6(Fr_damp_1)
  [Ff_damp_2] -> Load Transfer/7(Ff_damp_2)
  [Fr_damp_2] -> Load Transfer/8(Fr_damp_2)
  [Lt_f] -> Add13/1  "zr2"
  [Lt_r] -> Add13/2  "zr2"
  Add13/1 -> Scope6/1  "matlabFCN"
  [Lt_f] -> Lt_f/1  "zr2"
  [Lt_r] -> Lt_r/1  "zr2"

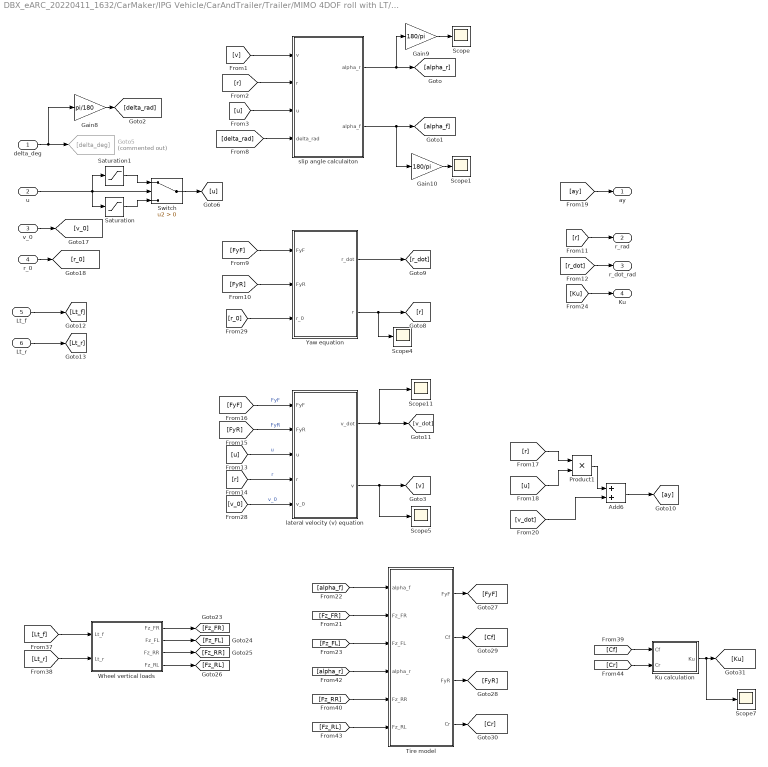
== system DBX_eARC_20220411_1632/CarMaker/IPG Vehicle/CarAndTrailer/Trailer/MIMO 4DOF roll with LT/Bicycle model ==
  delta_deg : Inport
  u : Inport  Port=2
  v_0 : Inport  Port=3
  r_0 : Inport  Port=4
  Lt_f : Inport  Port=5
  Lt_r : Inport  Port=6
  Add6 : Sum
  Gain10 : Gain  Gain=180/pi
  Gain8 : Gain  Gain=pi/180
  Gain9 : Gain  Gain=180/pi
  Goto5 : Goto  Commented=on  GotoTag=delta_deg
  Ku calculation : MATLAB Function  TreatAsAtomicUnit=on
  Product1 : Product
  Saturation : Saturate  UpperLimit=-eps  LowerLimit=-inf
  Saturation1 : Saturate  UpperLimit=inf  LowerLimit=eps
  Scope{,1,4..5,7,11} (6 alike) : Scope
  Switch : Switch  Criteria=u2 > Threshold
  Tire model : Subsystem
      settings: AttributesFormatString=%<MinAlgLoopOccurrences>
  Wheel vertical loads : Subsystem
      settings: AttributesFormatString=%<MinAlgLoopOccurrences>
  Yaw equation : Subsystem
  lateral velocity (v) equation : Subsystem
  slip angle calculaiton : Subsystem
  ay : Outport
  r_rad : Outport  Port=2
  r_dot_rad : Outport  Port=3
  Ku : Outport  Port=4
  wires:
  delta_deg/1 -> Gain8/1, Goto5/1
  [r] -> r_rad/1
  [r_dot] -> r_dot_rad/1
  [r] -> Product1/1
  [u] -> Product1/2
  [ay] -> ay/1
  Gain8/1 -> [delta_rad]
  Add6/1 -> [ay]
  Product1/1 -> Add6/1
  [v_dot] -> Add6/2
  Wheel vertical loads/4(Fz_RL) -> [Fz_RL]
  [Lt_f] -> Wheel vertical loads/1(Lt_f)
  [Lt_r] -> Wheel vertical loads/2(Lt_r)
  Wheel vertical loads/1(Fz_FR) -> [Fz_FR]
  Wheel vertical loads/3(Fz_RR) -> [Fz_RR]
  Wheel vertical loads/2(Fz_FL) -> [Fz_FL]
  Lt_f/1 -> [Lt_f]
  Lt_r/1 -> [Lt_r]
  [Fz_RR] -> Tire model/5(Fz_RR)
  Tire model/3(FyR) -> [FyR]
  Tire model/2(Cf) -> [Cf]
  Tire model/1(FyF) -> [FyF]
  [Fz_FL] -> Tire model/3(Fz_FL)
  [Fz_FR] -> Tire model/2(Fz_FR)
  [alpha_r] -> Tire model/4(alpha_r)
  Tire model/4(Cr) -> [Cr]
  [Fz_RL] -> Tire model/6(Fz_RL)
  [alpha_f] -> Tire model/1(alpha_f)
  [Cr] -> Ku calculation/2(Cr)
  [Cf] -> Ku calculation/1(Cf)
  Ku calculation/1(Ku) -> Scope7/1, [Ku]
  [Ku] -> Ku/1
  slip angle calculaiton/2(alpha_f) -> Gain10/1, [alpha_f]
  [r] -> slip angle calculaiton/2(r)
  [u] -> slip angle calculaiton/3(u)
  slip angle calculaiton/1(alpha_r) -> [alpha_r], Gain9/1
  Gain9/1 -> Scope/1
  [delta_rad] -> slip angle calculaiton/4(delta_rad)
  Gain10/1 -> Scope1/1
  [v] -> slip angle calculaiton/1(v)
  v_0/1 -> [v_0]
  r_0/1 -> [r_0]
  [r_0] -> Yaw equation/3(r_0)
  [FyR] -> Yaw equation/2(FyR)
  Yaw equation/1(r_dot) -> [r_dot]
  [FyF] -> Yaw equation/1(FyF)
  Yaw equation/2(r) -> [r], Scope4/1
  [FyR] -> lateral velocity (v) equation/2(FyR)  "FyR"
  [u] -> lateral velocity (v) equation/3(u)  "u"
  [FyF] -> lateral velocity (v) equation/1(FyF)  "FyF"
  [v_0] -> lateral velocity (v) equation/5(v_0)  "v_0"
  lateral velocity (v) equation/2(v) -> [v], Scope5/1
  lateral velocity (v) equation/1(v_dot) -> [v_dot], Scope11/1
  [r] -> lateral velocity (v) equation/4(r)  "r"
  Switch/1 -> [u]
  Saturation/1 -> Switch/3
  u/1 -> Saturation/1, Saturation1/1, Switch/2
  Saturation1/1 -> Switch/1
